simulink model "transformer_singlephase"  (R2014a)
settings: Solver=ode23tb  StartTime=0.0  StopTime=2/60  FixedStep=2e-6  MaxStep=1e-4  RelTol=1e-3
libraries: powerlib x7, simulink x1
settings Model: Creator=gdudgeon  LastModifiedBy=cosorio
settings DataIOCC: SignalLoggingSaveFormat=ModelDataLogs
settings OptimizationCC: ExpressionDepthLimit=2147483647
settings DebuggingCC: UnderspecifiedInitializationDetection=Classic  FcnCallInpInsideContextMsg=UseLocalSettings  UnconnectedLineMsg=none  StateNameClashWarn=warning
settings GRTTargetCC: CombineOutputUpdateFcns=off  GRTInterface=on

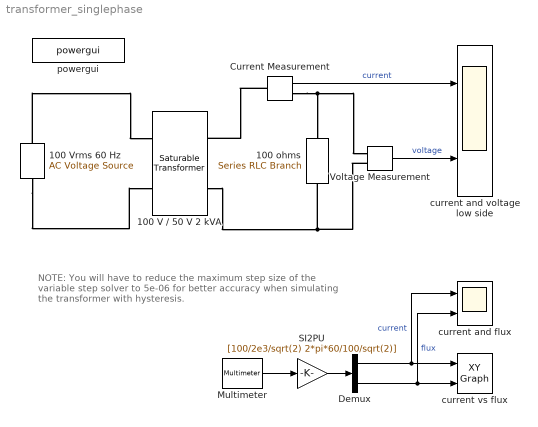
== system transformer_singlephase ==
  note: NOTE:
      | You will have to reduce the maximum step size of
      | the variable step solver to 5e-06 for better accuracy
      | when simulating the transformer with hysteresis.
  100 V / 50 V 2 kVA : powerlib/Elements/Saturable Transformer  ThreeWindings=off  Hysteresis=off  DataFile='hysteresis.mat'  Measurements=All measurements (V I Flux)  UNITS=pu  NominalPower=[2e3 60]  Winding1="[100  0.002 0.01]"  Winding2="[50  0.002 0.01]"  Winding3="[ 315e3  0.002  0.08 ]"  Saturation=[0,0 ; 0,1 ; 1.0,1.5 ]  CoreLoss=[500 -0.9]  MoreParameters=off  BreakLoop=on  DataType=off  InitialFlux=0  TransfoNumber=1
  100 Vrms 60 Hz : powerlib/Electrical Sources/AC Voltage Source  Amplitude=100*sqrt(2)  Phase=0  Frequency=60  SampleTime=0  Measurements=None
  100 ohms : powerlib/Elements/Series RLC Branch  LConnTagsString=__new0  RConnTagsString=__new0  BranchType=R  Resistance=100  Inductance=1e-3  SetiL0=off  InitialCurrent=0  Capacitance=1/2/pi  Setx0=off  InitialVoltage=0  Measurements=None
  Current Measurement : powerlib/Measurements/Current Measurement  PhasorSimulation=off  OutputType=Complex  PSBequivalent=0
  Demux : Demux  Outputs=2
  Multimeter : powerlib/Measurements/Multimeter  PhasorSimulation=off  OutputType=Complex  sel=[3 7]  L=7  Gain=[1 1]  yselected={'Iw1: Saturable Transformer 100 V // 50 V 2 kVA','Flux: Saturable Transformer 100 V // 50 V 2 kVA'};  PSBOutputType=1  PSBequivalent=0  AxesSetting=[0,0.1,-100,100]  Display=0  SavedBlockNames=-11
  SI2PU : Gain  Gain=[100/2e3/sqrt(2) 2*pi*60/100/sqrt(2)]
  Voltage Measurement : powerlib/Measurements/Voltage Measurement  PhasorSimulation=off  OutputType=Complex  PSBequivalent=0
  current and flux : Scope  NumInputPorts=2
      settings: YMin=-0.025~-1  YMax=0.2~1.25  SaveName=current_flux
  current and voltage low side : Scope  NumInputPorts=2
      settings: YMin=-1~-100  YMax=1~100  SaveName=current_flux1
  current vs flux : simulink/Sinks/XY Graph  xmin=-2  xmax=2  ymin=-1.5  ymax=1.5  st=-1
  powergui : powerlib/powergui  SimulationMode=Continuous  SolverType=Tustin  SampleTime=5e-6  frequency=60  SPID=off  DisableSnubberDevices=off  DisableRonSwitches=off  DisableVfSwitches=off  SwTol=0  Interpol=off  DisplayEquations=off  Ts=0  methode=off  frequencyindice=60  Pbase=100e6  ErrMax=1e-4  Iterations=50  UnitsV=kV  UnitsW=MW  FunctionMessages=off  echomessages=off  HookPort=off  EnableUseOfTLC=off  x0status=blocks  RestoreLinks=warning  ResistiveCurrentMeasurement=off  Frange=[0.1:0.02:100]  Ylog=off  Xlog=on  ShowGrid=on  save=off  variable=ZData  structure=VC  ZoomFFT=off  StartTime=0.0  cycles=1  DisplayStyle=1  fundamental=60  FreqAxis=off  MaxFrequency=1000  frequencyindicesteady=1  RmsSteady=1  display=off
  wires:
  Current Measurement/1 -> current and voltage low side/1  "current"
  Voltage Measurement/1 -> current and voltage low side/2  "voltage"
  Multimeter/1 -> SI2PU/1
  Demux/1 -> current vs flux/1, current and flux/1  "current"
  Demux/2 -> current vs flux/2, current and flux/2  "flux"
  SI2PU/1 -> Demux/1
  connections:
  Current Measurement/LConn1 -- 100 V / 50 V 2 kVA/RConn1
  100 V / 50 V 2 kVA/RConn2 -- Voltage Measurement/LConn2 -- 100 ohms/RConn1
  Current Measurement/RConn1 -- Voltage Measurement/LConn1 -- 100 ohms/LConn1
  100 Vrms 60 Hz/LConn1 -- 100 V / 50 V 2 kVA/LConn2
  100 Vrms 60 Hz/RConn1 -- 100 V / 50 V 2 kVA/LConn1
